simulink model "BPSK_modulation"  (Simulink 10.2)
settings: Solver=ode45  StartTime=0.0  StopTime=10.0  RelTol=1e-3  EnableMultiTasking=on
libraries: commrandsrc2 x1
settings Model: Creator=User  LastModifiedBy=HP
settings DataIOCC: LimitDataPoints=on  SignalLoggingSaveFormat=Dataset
settings DebuggingCC: SolverPrmCheckMsg=warning  FcnCallInpInsideContextMsg=error  StateNameClashWarn=warning
settings GRTTargetCC: CombineOutputUpdateFcns=on  GRTInterface=off
settings SimscapeCC: SimscapeNormalizeSystem=off

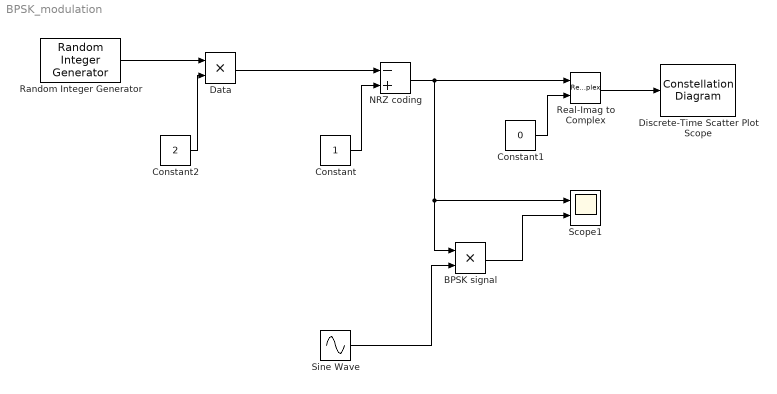
== system BPSK_modulation ==
  BPSK signal : Product
  Constant : Constant
  Constant1 : Constant  Value=0
  Constant2 : Constant  Value=2
  Data : Product
  Discrete-Time Scatter Plot Scope : ConstellationDiagram  Tag=ScatterPlot
  NRZ coding : Sum  Inputs=-+
  Random Integer Generator : commrandsrc2/Random Integer Generator  mul=2  seed=37  Ts=1/10  frameBased=off  sampPerFrame=1  orient=off  outDataType=double
      settings: SourceProductBaseCode=CM
  Real-Imag to Complex : RealImagToComplex
  Scope1 : Scope  NumInputPorts=2
  Sine Wave : Sin  Frequency=60*pi  Phase=pi/2  SampleTime=0.001
  wires:
  Sine Wave/1 -> BPSK signal/2
  Real-Imag to Complex/1 -> Discrete-Time Scatter Plot Scope/1
  BPSK signal/1 -> Scope1/2
  Constant1/1 -> Real-Imag to Complex/2
  Random Integer Generator/1 -> Data/1
  Constant2/1 -> Data/2
  Data/1 -> NRZ coding/1
  Constant/1 -> NRZ coding/2
  NRZ coding/1 -> Scope1/1, BPSK signal/1, Real-Imag to Complex/1
